simulink model "Model"  (R2016b)
settings: Solver=VariableStepAuto  StartTime=0.0  StopTime=20  RelTol=1e-3
values from neighbouring files (symbols this model uses):
  dpitch = 7.203    [Parameters.m]
  droll = 0.1094    [Parameters.m]
  dx = 2.86    [Parameters.m]
  dyaw = 0.26285    [Parameters.m]
  dz = 0    [Parameters.m]
  Ix = 0.06541    [Parameters.m]
  Iy = 1.08921    [Parameters.m]
  Iz = 1.10675    [Parameters.m]
  l1 = 0.05    [Parameters.m]
  l2 = 0.05    [Parameters.m]
  Tpitch = 131.8316    [Parameters.m]
  Troll = 6.9736    [Parameters.m]
undefined symbols (not defined in the file or in its folder): F1, F2, m
settings Model: Creator=USUARIO  LastModifiedBy=USUARIO
settings DataIOCC: Refine=100

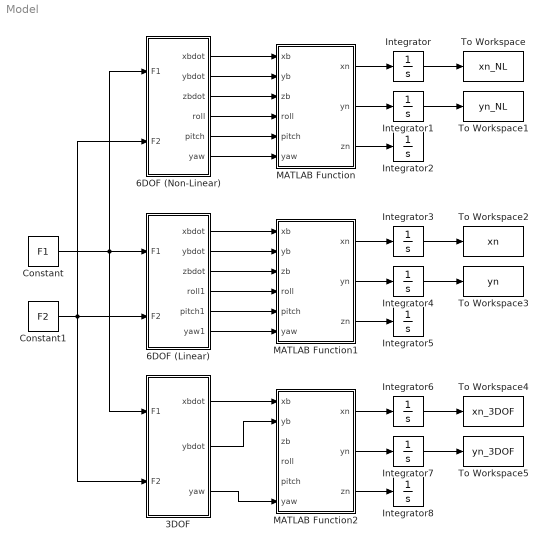
== system Model ==
  3DOF : Subsystem
  6DOF (Linear) : Subsystem
  6DOF (Non-Linear) : Subsystem
  Constant : Constant  Value=F1
  Constant1 : Constant  Value=F2
  Integrator{,1..8} (9 alike) : Integrator
  MATLAB Function : MATLAB Function  TreatAsAtomicUnit=on
  MATLAB Function1 : MATLAB Function  TreatAsAtomicUnit=on
  MATLAB Function2 : MATLAB Function  TreatAsAtomicUnit=on
  To Workspace : ToWorkspace  VariableName=xn_NL  SaveFormat=Timeseries  SampleTime=-1
  To Workspace1 : ToWorkspace  VariableName=yn_NL  SaveFormat=Timeseries  SampleTime=-1
  To Workspace2 : ToWorkspace  VariableName=xn  SaveFormat=Timeseries  SampleTime=-1
  To Workspace3 : ToWorkspace  VariableName=yn  SaveFormat=Timeseries  SampleTime=-1
  To Workspace4 : ToWorkspace  VariableName=xn_3DOF  SaveFormat=Timeseries  SampleTime=-1
  To Workspace5 : ToWorkspace  VariableName=yn_3DOF  SaveFormat=Timeseries  SampleTime=-1
  wires:
  Constant/1 -> 6DOF (Non-Linear)/1(F1), 6DOF (Linear)/1(F1), 3DOF/1(F1)
  Constant1/1 -> 6DOF (Non-Linear)/2(F2), 6DOF (Linear)/2(F2), 3DOF/2(F2)
  MATLAB Function/1(xn) -> Integrator/1
  MATLAB Function/2(yn) -> Integrator1/1
  6DOF (Non-Linear)/6(yaw) -> MATLAB Function/6(yaw)
  6DOF (Non-Linear)/5(pitch) -> MATLAB Function/5(pitch)
  6DOF (Non-Linear)/4(roll) -> MATLAB Function/4(roll)
  6DOF (Non-Linear)/3(zbdot) -> MATLAB Function/3(zb)
  6DOF (Non-Linear)/2(ybdot) -> MATLAB Function/2(yb)
  6DOF (Non-Linear)/1(xbdot) -> MATLAB Function/1(xb)
  3DOF/1(xbdot) -> MATLAB Function2/1(xb)
  3DOF/2(ybdot) -> MATLAB Function2/2(yb)
  3DOF/3(yaw) -> MATLAB Function2/6(yaw)
  MATLAB Function1/1(xn) -> Integrator3/1
  MATLAB Function1/2(yn) -> Integrator4/1
  MATLAB Function/3(zn) -> Integrator2/1
  Integrator/1 -> To Workspace/1
  Integrator1/1 -> To Workspace1/1
  6DOF (Linear)/1(xbdot) -> MATLAB Function1/1(xb)
  6DOF (Linear)/2(ybdot) -> MATLAB Function1/2(yb)
  6DOF (Linear)/3(zbdot) -> MATLAB Function1/3(zb)
  6DOF (Linear)/4(roll1) -> MATLAB Function1/4(roll)
  6DOF (Linear)/5(pitch1) -> MATLAB Function1/5(pitch)
  6DOF (Linear)/6(yaw1) -> MATLAB Function1/6(yaw)
  Integrator3/1 -> To Workspace2/1
  Integrator4/1 -> To Workspace3/1
  MATLAB Function1/3(zn) -> Integrator5/1
  MATLAB Function2/1(xn) -> Integrator6/1
  MATLAB Function2/2(yn) -> Integrator7/1
  Integrator6/1 -> To Workspace4/1
  Integrator7/1 -> To Workspace5/1
  MATLAB Function2/3(zn) -> Integrator8/1

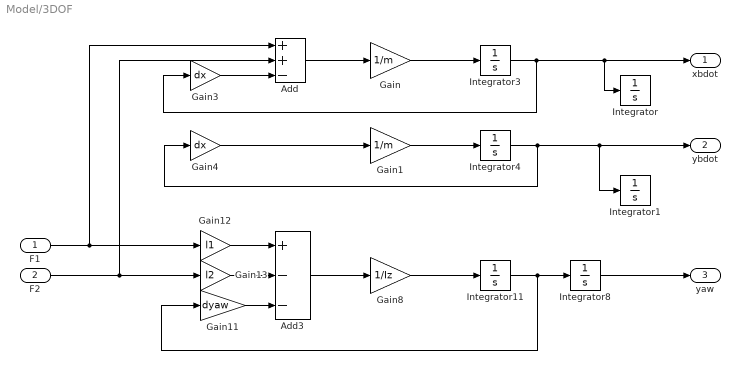
== system Model/3DOF ==
  F1 : Inport
  F2 : Inport  Port=2
  Add : Sum  Inputs=++-
  Add3 : Sum  Inputs=+--
  Gain : Gain  Gain=1/m
  Gain1 : Gain  Gain=1/m
  Gain11 : Gain  Gain=dyaw
  Gain12 : Gain  Gain=l1
  Gain13 : Gain  Gain=l2
  Gain3 : Gain  Gain=dx
  Gain4 : Gain  Gain=dx
  Gain8 : Gain  Gain=1/Iz
  Integrator{,1,3..4,8,11} (6 alike) : Integrator
  xbdot : Outport
  ybdot : Outport  Port=2
  yaw : Outport  Port=3
  wires:
  F1/1 -> Add/1, Gain12/1
  Integrator11/1 -> Gain11/1, Integrator8/1
  Gain8/1 -> Integrator11/1
  Gain4/1 -> Gain1/1
  Gain1/1 -> Integrator4/1
  Gain3/1 -> Add/3
  F2/1 -> Gain13/1, Add/2
  Add/1 -> Gain/1
  Gain/1 -> Integrator3/1
  Gain12/1 -> Add3/1
  Add3/1 -> Gain8/1
  Gain11/1 -> Add3/3
  Gain13/1 -> Add3/2
  Integrator3/1 -> Integrator/1, xbdot/1, Gain3/1
  Integrator4/1 -> Integrator1/1, ybdot/1, Gain4/1
  Integrator8/1 -> yaw/1

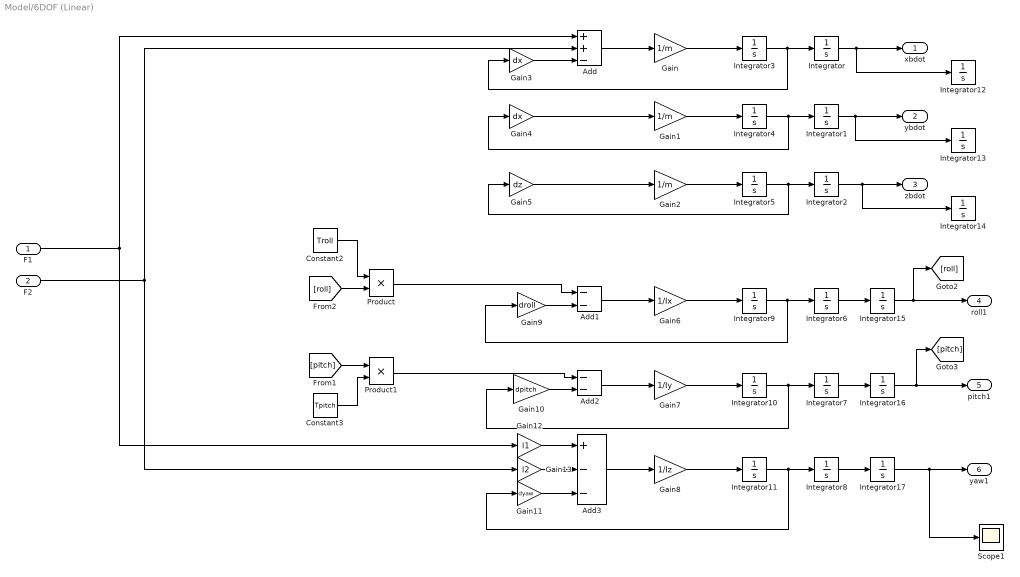
== system Model/6DOF (Linear) ==
  F1 : Inport
  F2 : Inport  Port=2
  Add : Sum  Inputs=++-
  Add1 : Sum  Inputs=--
  Add2 : Sum  Inputs=--
  Add3 : Sum  Inputs=+--
  Constant2 : Constant  Value=Troll
  Constant3 : Constant  Value=Tpitch
  Gain : Gain  Gain=1/m
  Gain1 : Gain  Gain=1/m
  Gain10 : Gain  Gain=dpitch
  Gain11 : Gain  Gain=dyaw
  Gain12 : Gain  Gain=l1
  Gain13 : Gain  Gain=l2
  Gain2 : Gain  Gain=1/m
  Gain3 : Gain  Gain=dx
  Gain4 : Gain  Gain=dx
  Gain5 : Gain  Gain=dz
  Gain6 : Gain  Gain=1/Ix
  Gain7 : Gain  Gain=1/Iy
  Gain8 : Gain  Gain=1/Iz
  Gain9 : Gain  Gain=droll
  Integrator{,1..17} (18 alike) : Integrator
  Product : Product
  Product1 : Product
  Scope1 : Scope
  xbdot : Outport
  ybdot : Outport  Port=2
  zbdot : Outport  Port=3
  roll1 : Outport  Port=4
  pitch1 : Outport  Port=5
  yaw1 : Outport  Port=6
  wires:
  Product/1 -> Add1/1
  Product1/1 -> Add2/1
  Gain9/1 -> Add1/2
  Gain13/1 -> Add3/2
  Gain11/1 -> Add3/3
  Add3/1 -> Gain8/1
  Constant2/1 -> Product/1
  Gain12/1 -> Add3/1
  Constant3/1 -> Product1/2
  Gain10/1 -> Add2/2
  Add2/1 -> Gain7/1
  Add1/1 -> Gain6/1
  Integrator6/1 -> Integrator15/1
  Integrator4/1 -> Integrator1/1, Gain4/1
  Gain/1 -> Integrator3/1
  Add/1 -> Gain/1
  F2/1 -> Add/2, Gain13/1
  Gain2/1 -> Integrator5/1
  Gain3/1 -> Add/3
  Gain1/1 -> Integrator4/1
  Gain5/1 -> Gain2/1
  Gain4/1 -> Gain1/1
  Integrator10/1 -> Integrator7/1, Gain10/1
  Gain8/1 -> Integrator11/1
  Integrator11/1 -> Integrator8/1, Gain11/1
  Gain7/1 -> Integrator10/1
  Gain6/1 -> Integrator9/1
  Integrator9/1 -> Integrator6/1, Gain9/1
  Integrator5/1 -> Integrator2/1, Gain5/1
  F1/1 -> Add/1, Gain12/1
  Integrator3/1 -> Integrator/1, Gain3/1
  [roll] -> Product/2
  [pitch] -> Product1/1
  Integrator2/1 -> Integrator14/1, zbdot/1
  Integrator17/1 -> Scope1/1, yaw1/1
  Integrator16/1 -> pitch1/1, [pitch]
  Integrator15/1 -> roll1/1, [roll]
  Integrator/1 -> Integrator12/1, xbdot/1
  Integrator1/1 -> Integrator13/1, ybdot/1
  Integrator7/1 -> Integrator16/1
  Integrator8/1 -> Integrator17/1

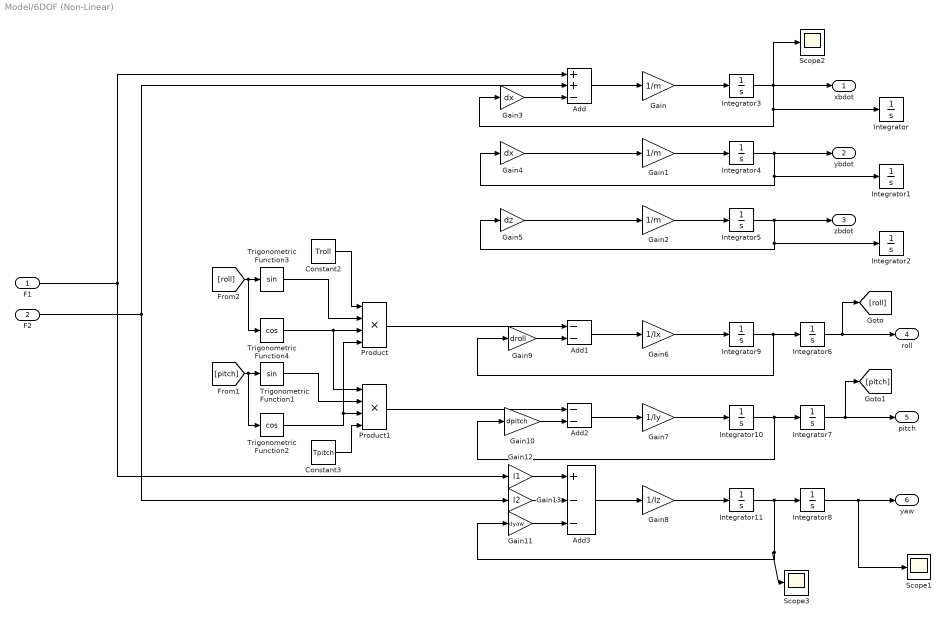
== system Model/6DOF (Non-Linear) ==
  F1 : Inport
  F2 : Inport  Port=2
  Add : Sum  Inputs=++-
  Add1 : Sum  Inputs=--
  Add2 : Sum  Inputs=--
  Add3 : Sum  Inputs=+--
  Constant2 : Constant  Value=Troll
  Constant3 : Constant  Value=Tpitch
  Gain : Gain  Gain=1/m
  Gain1 : Gain  Gain=1/m
  Gain10 : Gain  Gain=dpitch
  Gain11 : Gain  Gain=dyaw
  Gain12 : Gain  Gain=l1
  Gain13 : Gain  Gain=l2
  Gain2 : Gain  Gain=1/m
  Gain3 : Gain  Gain=dx
  Gain4 : Gain  Gain=dx
  Gain5 : Gain  Gain=dz
  Gain6 : Gain  Gain=1/Ix
  Gain7 : Gain  Gain=1/Iy
  Gain8 : Gain  Gain=1/Iz
  Gain9 : Gain  Gain=droll
  Integrator{,1..11} (12 alike) : Integrator
  Product : Product  Inputs=4
  Product1 : Product  Inputs=4
  Scope1 : Scope
  Scope2 : Scope
  Scope3 : Scope
  Trigonometric Function1 : Trigonometry
  Trigonometric Function2 : Trigonometry  Operator=cos
  Trigonometric Function3 : Trigonometry
  Trigonometric Function4 : Trigonometry  Operator=cos
  xbdot : Outport
  ybdot : Outport  Port=2
  zbdot : Outport  Port=3
  roll : Outport  Port=4
  pitch : Outport  Port=5
  yaw : Outport  Port=6
  wires:
  F1/1 -> Gain12/1, Add/1
  Gain6/1 -> Integrator9/1
  Gain7/1 -> Integrator10/1
  Gain8/1 -> Integrator11/1
  Gain4/1 -> Gain1/1
  Gain5/1 -> Gain2/1
  Gain1/1 -> Integrator4/1
  Gain3/1 -> Add/3
  Gain2/1 -> Integrator5/1
  F2/1 -> Gain13/1, Add/2
  Add/1 -> Gain/1
  Gain/1 -> Integrator3/1
  Integrator9/1 -> Integrator6/1, Gain9/1
  Integrator10/1 -> Integrator7/1, Gain10/1
  Add1/1 -> Gain6/1
  Add2/1 -> Gain7/1
  Gain10/1 -> Add2/2
  Constant3/1 -> Product1/4
  Gain12/1 -> Add3/1
  Constant2/1 -> Product/1
  Add3/1 -> Gain8/1
  Gain11/1 -> Add3/3
  Gain13/1 -> Add3/2
  Gain9/1 -> Add1/2
  Product1/1 -> Add2/1
  Trigonometric Function4/1 -> Product1/1, Product/3
  Trigonometric Function1/1 -> Product1/2
  [pitch] -> Trigonometric Function2/1, Trigonometric Function1/1
  Trigonometric Function2/1 -> Product1/3, Product/4
  [roll] -> Trigonometric Function4/1, Trigonometric Function3/1
  Product/1 -> Add1/1
  Trigonometric Function3/1 -> Product/2
  Integrator5/1 -> zbdot/1, Integrator2/1, Gain5/1
  Integrator11/1 -> Integrator8/1, Scope3/1, Gain11/1
  Integrator8/1 -> Scope1/1, yaw/1
  Integrator7/1 -> pitch/1, [pitch]
  Integrator6/1 -> roll/1, [roll]
  Integrator3/1 -> xbdot/1, Scope2/1, Integrator/1, Gain3/1
  Integrator4/1 -> ybdot/1, Integrator1/1, Gain4/1

== matlab function Model/MATLAB Function1 ==
  data: xb input; xn output; yb input; zb input; roll input; pitch input; yaw input; yn output; zn output
function [xn,yn,zn] = fcn(xb,yb,zb,roll,pitch,yaw)
R=[cos(pitch)*cos(yaw) sin(roll)*sin(pitch)*cos(yaw)-cos(roll)*sin(yaw) ...
                          cos(roll)*sin(pitch)*cos(yaw)+sin(roll)*sin(yaw);
   cos(pitch)*sin(yaw) sin(roll)*sin(pitch)*sin(yaw)+cos(roll)*cos(yaw) ...
                          cos(roll)*sin(pitch)*sin(yaw)-sin(roll)*cos(yaw);
   -sin(pitch) sin(roll)*cos(pitch) cos(roll)*cos(pitch)];

n=R*[xb;yb;zb];

xn=n(1);
yn=n(2);
zn=n(3);
end

== matlab function Model/MATLAB Function ==
  data: xb input; xn output; yb input; zb input; roll input; pitch input; yaw input; yn output; zn output
function [xn,yn,zn] = fcn(xb,yb,zb,roll,pitch,yaw)
R=[cos(pitch)*cos(yaw) sin(roll)*sin(pitch)*cos(yaw)-cos(roll)*sin(yaw) ...
                          cos(roll)*sin(pitch)*cos(yaw)+sin(roll)*sin(yaw);
   cos(pitch)*sin(yaw) sin(roll)*sin(pitch)*sin(yaw)+cos(roll)*cos(yaw) ...
                          cos(roll)*sin(pitch)*sin(yaw)-sin(roll)*cos(yaw);
   -sin(pitch) sin(roll)*cos(pitch) cos(roll)*cos(pitch)];

n=R*[xb;yb;zb];

xn=n(1);
yn=n(2);
zn=n(3);
end

== matlab function Model/MATLAB Function2 ==
  data: xb input; xn output; yb input; zb input; roll input; pitch input; yaw input; yn output; zn output
function [xn,yn,zn] = fcn(xb,yb,zb,roll,pitch,yaw)
R=[cos(pitch)*cos(yaw) sin(roll)*sin(pitch)*cos(yaw)-cos(roll)*sin(yaw) ...
                          cos(roll)*sin(pitch)*cos(yaw)+sin(roll)*sin(yaw);
   cos(pitch)*sin(yaw) sin(roll)*sin(pitch)*sin(yaw)+cos(roll)*cos(yaw) ...
                          cos(roll)*sin(pitch)*sin(yaw)-sin(roll)*cos(yaw);
   -sin(pitch) sin(roll)*cos(pitch) cos(roll)*cos(pitch)];

n=R*[xb;yb;zb];

xn=n(1);
yn=n(2);
zn=n(3);
end
